simulink model "Lane_Keeping_control_BMW730_auto_sim"  (R2021a)
settings: Solver=FixedStepAuto  StartTime=0.0  StopTime=time  FixedStep=step_size  RelTol=1e-3
values from neighbouring files (symbols this model uses):
  alpha = cf/m+cr/m    (= 169.206008584)    [Dynamic_steering.m]    (also in Dynamic_steering_control_5_1.m; Dynamic_steering_control_5_1_cycle.m; Lane_Keeping_control_BMW730.m)
  alpha_r = alpha    (= 169.206008584)    [Lane_Keeping_control_BMW730.m]
  b1 = cf/m    (= 54.5064377682)    [Dynamic_steering.m]    (also in Dynamic_steering_control_5_1.m; Dynamic_steering_control_5_1_cycle.m; Lane_Keeping_control_BMW730.m)
  b1_r = b1    (= 54.5064377682)    [Lane_Keeping_control_BMW730.m]
  b2 = cf*lf/J    (= 41.9857690203)    [Dynamic_steering.m]    (also in Dynamic_steering_control_5_1.m; Dynamic_steering_control_5_1_cycle.m; Lane_Keeping_control_BMW730.m)
  b2_r = b2    (= 41.9857690203)    [Lane_Keeping_control_BMW730.m]
  beta = -cf*lf+cr*lr    (= 128800)    [Dynamic_steering.m]    (also in Dynamic_steering_control_5_1.m; Dynamic_steering_control_5_1_cycle.m; Lane_Keeping_control_BMW730.m)
  beta_r = beta    (= 128800)    [Lane_Keeping_control_BMW730.m]
  dC = double(dC)    [HM8_Youla.m]    (also in Lane_Keeping_control_BMW730.m)
  gamma = 0.01    [Cart_pendulum.m]    (also in Dynamic_steering.m = 165.348461959; Dynamic_steering_control_5_1.m = 165.348461959; Dynamic_steering_control_5_1_cycle.m = 165.348461959; Lane_Keeping_control_BMW730.m = 165.348461959)
  gamma_r = gamma    (= 165.348461959)    [Lane_Keeping_control_BMW730.m]
  J = 100    [Cart_pendulum.m]    (also in Dynamic_steering.m = 3654; Dynamic_steering_control_5_1.m = 3654; Dynamic_steering_control_5_1_cycle.m = 3654; Lane_Keeping_control_BMW730.m = 3654)
  kd = -1    [Lane_Keeping_control_BMW730.m]
  kI2 = -0.01    [Lane_Keeping_control_BMW730.m]
  kI3 = -0.1    [Lane_Keeping_control_BMW730.m]
  kP2 = -10    [Lane_Keeping_control_BMW730.m]
  m = 50    [Active_suspension_with_control_2.m]    (also in Cart_pendulum.m = 80; Dynamic_steering.m = 1864; Dynamic_steering_control_5_1.m = 1864; Dynamic_steering_control_5_1_cycle.m = 1864)
  nC = double(nC)    [HM8_Youla.m]    (also in Lane_Keeping_control_BMW730.m)
  r = 100    [Lane_Keeping_control_BMW730.m]
  V = Vzf1(2)    [Dynamic_steering.m]    (also in Dynamic_steering_control_5_1.m = 33.3333333333; Dynamic_steering_control_5_1_cycle.m = ( V0/3.6 )*( 1+ i/100 ); Lane_Keeping_control_BMW730.m = 17)
  vy_0 = 2    [Dynamic_steering_control_5_1.m]    (also in Dynamic_steering_control_5_1_cycle.m; Lane_Keeping_control_BMW730.m = 0)
  vy_r0 = 0    [Lane_Keeping_control_BMW730.m]
libraries: simulink x3
settings Model: Creator=Gerardo  LastModifiedBy=adith
settings SolverCC: AlgebraicLoopSolver=TrustRegion
settings DataIOCC: ReturnWorkspaceOutputs=off
settings DebuggingCC: SFMachineParentedDataDiag=warning  ArithmeticOperatorsInVariantConditions=warning
settings SFSimCC: CustomCodeUndefinedFunction=UseInterfaceOnly

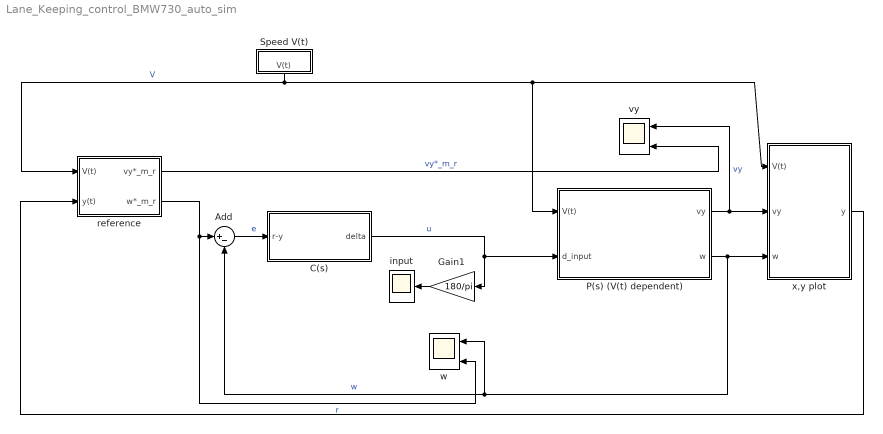
== system Lane_Keeping_control_BMW730_auto_sim ==
  Add : Sum  Inputs=|+-
  C(s) : Subsystem
  Gain1 : Gain  Gain=180/pi
  P(s) (V(t) dependent) : Subsystem
  Speed V(t) : Subsystem
  input : Scope
  reference : Subsystem
  vy : Scope  NumInputPorts=2
  w : Scope  NumInputPorts=2
  x,y plot : Subsystem
  wires:
  C(s)/1(delta) -> P(s) (V(t) dependent)/2(d_input), Gain1/1  "u"
  Add/1 -> C(s)/1(r-y)  "e"
  P(s) (V(t) dependent)/2(w) -> w/1, Add/2, x,y plot/3(w)  "w"
  reference/2(w*_m_r) -> w/2, Add/1  "r"
  P(s) (V(t) dependent)/1(vy) -> x,y plot/2(vy), vy/1  "vy"
  reference/1(vy*_m_r) -> vy/2  "vy*_m_r"
  Speed V(t)/1(V(t)) -> reference/1(V(t)), P(s) (V(t) dependent)/1(V(t)), x,y plot/1(V(t))  "V"
  Gain1/1 -> input/1
  x,y plot/1(y) -> reference/2(y(t))

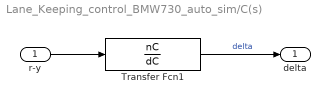
== system Lane_Keeping_control_BMW730_auto_sim/C(s) ==
  r-y : Inport
  Transfer Fcn1 : TransferFcn  Numerator=nC  Denominator=dC
  delta : Outport  VectorParamsAs1DForOutWhenUnconnected=off
  wires:
  Transfer Fcn1/1 -> delta/1  "delta"
  r-y/1 -> Transfer Fcn1/1

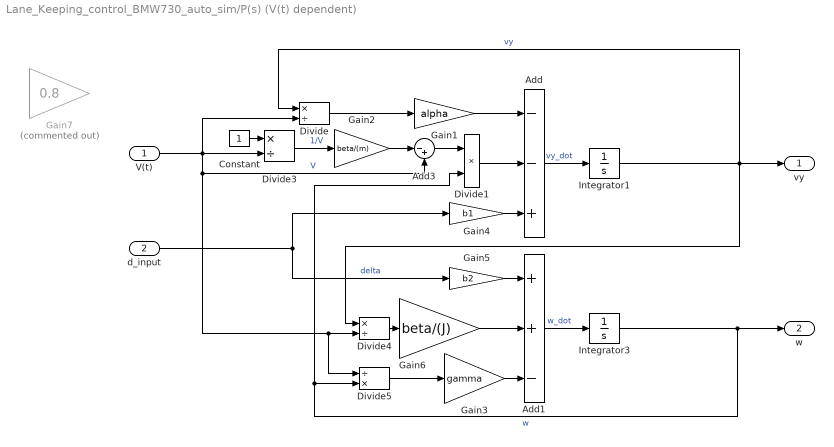
== system Lane_Keeping_control_BMW730_auto_sim/P(s) (V(t) dependent) ==
  V(t) : Inport
  d_input : Inport  Port=2
  Add : Sum  Inputs=--+
  Add1 : Sum  Inputs=++-
  Add3 : Sum  Inputs=|-+
  Constant : Constant
  Divide : Product  Inputs=*/
  Divide1 : Product  Inputs=**
  Divide3 : Product  Inputs=*/
  Divide4 : Product  Inputs=*/
  Divide5 : Product  Inputs=/*
  Gain1 : Gain  Gain=alpha
  Gain2 : Gain  Gain=beta/(m)
  Gain3 : Gain  Gain=gamma
  Gain4 : Gain  Gain=b1
  Gain5 : Gain  Gain=b2
  Gain6 : Gain  Gain=beta/(J)
  Gain7 : Gain  Commented=on  Gain=0.8
  Integrator1 : Integrator  InitialCondition=vy_0
  Integrator3 : Integrator
  vy : Outport  VectorParamsAs1DForOutWhenUnconnected=off
  w : Outport  Port=2  VectorParamsAs1DForOutWhenUnconnected=off
  wires:
  Gain3/1 -> Add1/3
  Add/1 -> Integrator1/1  "vy_dot"
  Add1/1 -> Integrator3/1  "w_dot"
  Gain1/1 -> Add/1
  Gain5/1 -> Add1/1
  Gain4/1 -> Add/3
  Gain2/1 -> Add3/1
  Integrator1/1 -> Divide4/1, Divide/1, vy/1  "vy"
  Divide5/1 -> Gain3/1
  V(t)/1 -> Divide3/2, Divide5/1, Divide4/2, Add3/2, Divide/2  "V"
  Divide3/1 -> Gain2/1  "1/V"
  d_input/1 -> Gain4/1, Gain5/1  "delta"
  Divide4/1 -> Gain6/1
  Gain6/1 -> Add1/2
  Divide1/1 -> Add/2
  Divide/1 -> Gain1/1
  Integrator3/1 -> Divide5/2, Divide1/2, w/1  "w"
  Constant/1 -> Divide3/1
  Add3/1 -> Divide1/1

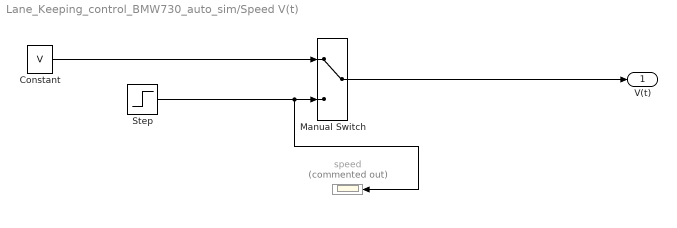
== system Lane_Keeping_control_BMW730_auto_sim/Speed V(t) ==
  Constant : Constant  Value=V
  Manual Switch : ManualSwitch
  Step : Step  Time=7.5  Before=V  After=V*0.85  SampleTime=0
  speed : Scope  Commented=on
  V(t) : Outport  VectorParamsAs1DForOutWhenUnconnected=off
  wires:
  Constant/1 -> Manual Switch/1
  Step/1 -> speed/1, Manual Switch/2
  Manual Switch/1 -> V(t)/1

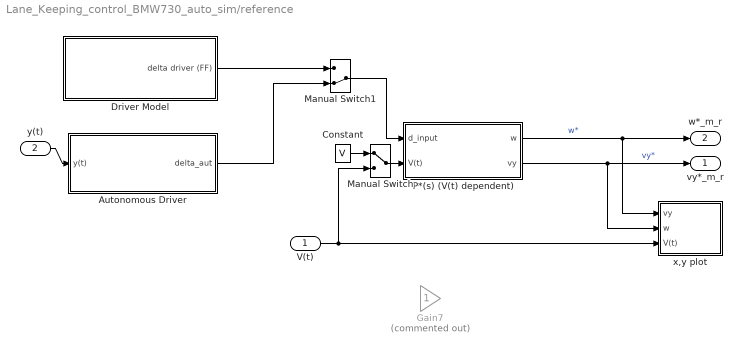
== system Lane_Keeping_control_BMW730_auto_sim/reference ==
  V(t) : Inport
  y(t) : Inport  Port=2
  Autonomous Driver : Subsystem
  Constant : Constant  Value=V
  Driver Model : Subsystem
  Gain7 : Gain  Commented=on
  Manual Switch : ManualSwitch
  Manual Switch1 : ManualSwitch  CurrentSetting=0
  P*(s) (V(t) dependent) : Subsystem
  x,y plot : Subsystem
  vy*_m_r : Outport  VectorParamsAs1DForOutWhenUnconnected=off
  w*_m_r : Outport  Port=2  VectorParamsAs1DForOutWhenUnconnected=off
  wires:
  P*(s) (V(t) dependent)/1(w) -> x,y plot/1(vy), w*_m_r/1  "w*"
  P*(s) (V(t) dependent)/2(vy) -> x,y plot/2(w), vy*_m_r/1  "vy*"
  Manual Switch/1 -> P*(s) (V(t) dependent)/2(V(t))
  Constant/1 -> Manual Switch/1
  V(t)/1 -> Manual Switch/2, x,y plot/3(V(t))
  Manual Switch1/1 -> P*(s) (V(t) dependent)/1(d_input)
  Driver Model/1(delta driver (FF)) -> Manual Switch1/1
  Autonomous Driver/1(delta_aut) -> Manual Switch1/2
  y(t)/1 -> Autonomous Driver/1(y(t))

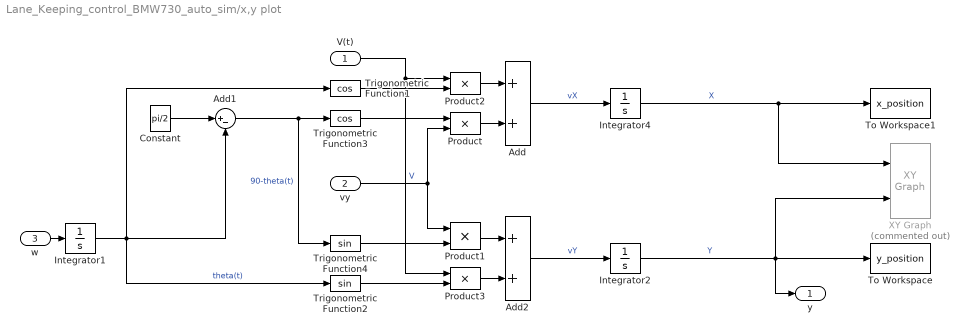
== system Lane_Keeping_control_BMW730_auto_sim/x,y plot ==
  V(t) : Inport
  vy : Inport  Port=2
  w : Inport  Port=3
  Add : Sum
  Add1 : Sum  Inputs=|+-
  Add2 : Sum
  Constant : Constant  Value=pi/2
  Integrator1 : Integrator
  Integrator2 : Integrator
  Integrator4 : Integrator
  Product{,1..3} (4 alike) : Product
  To Workspace : ToWorkspace  VariableName=y_position  SampleTime=-1
      settings: Save2DSignal=2-D array (concatenate along first dimension)
  To Workspace1 : ToWorkspace  VariableName=x_position  SampleTime=-1
      settings: Save2DSignal=2-D array (concatenate along first dimension)
  Trigonometric Function1 : Trigonometry  Operator=cos
  Trigonometric Function2 : Trigonometry
  Trigonometric Function3 : Trigonometry  Operator=cos
  Trigonometric Function4 : Trigonometry
  XY Graph : simulink/Sinks/XY Graph  Commented=on  xmin=-1000  xmax=1000  ymin=-50  ymax=50  st=-1
  y : Outport  VectorParamsAs1DForOutWhenUnconnected=off
  wires:
  Trigonometric Function4/1 -> Product1/2
  Trigonometric Function3/1 -> Product/1
  Product1/1 -> Add2/1
  Trigonometric Function2/1 -> Product3/2
  Add2/1 -> Integrator2/1  "vY"
  Trigonometric Function1/1 -> Product2/2
  Product/1 -> Add/2
  Add1/1 -> Trigonometric Function3/1, Trigonometric Function4/1  "90-theta(t)"
  Integrator1/1 -> Trigonometric Function1/1, Trigonometric Function2/1, Add1/2  "theta(t)"
  w/1 -> Integrator1/1
  Constant/1 -> Add1/1
  Add/1 -> Integrator4/1  "vX"
  Integrator4/1 -> XY Graph/1, To Workspace1/1  "X"
  vy/1 -> Product/2, Product1/1
  Integrator2/1 -> y/1, To Workspace/1, XY Graph/2  "Y"
  Product2/1 -> Add/1
  V(t)/1 -> Product3/1, Product2/1  "V"
  Product3/1 -> Add2/2

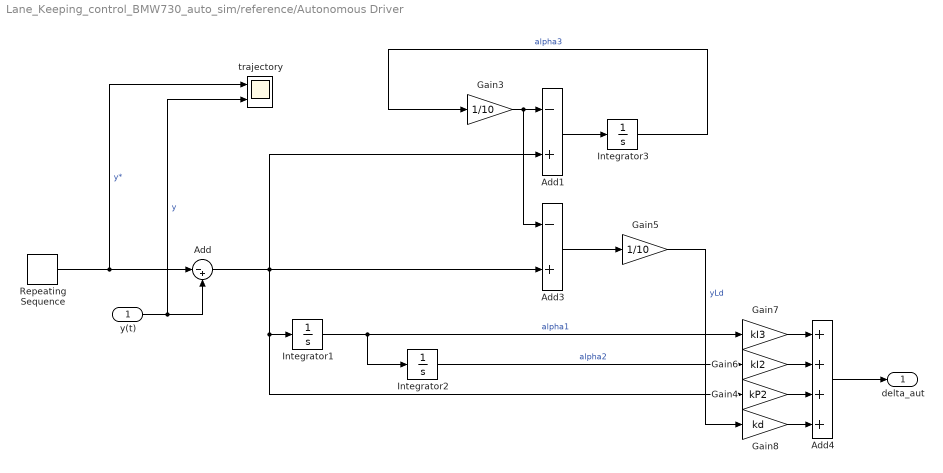
== system Lane_Keeping_control_BMW730_auto_sim/reference/Autonomous Driver ==
  y(t) : Inport
  Add : Sum  Inputs=|-+
  Add1 : Sum  Inputs=-+
  Add3 : Sum  Inputs=-+
  Add4 : Sum  Inputs=++++
  Gain3 : Gain  Gain=1/10
  Gain4 : Gain  Gain=kP2
  Gain5 : Gain  Gain=1/10
  Gain6 : Gain  Gain=kI2
  Gain7 : Gain  Gain=kI3
  Gain8 : Gain  Gain=kd
  Integrator1 : Integrator
  Integrator2 : Integrator
  Integrator3 : Integrator
  Repeating Sequence : simulink/Sources/Repeating Sequence  rep_seq_t=t  rep_seq_y=y_position
  trajectory : Scope  NumInputPorts=2
  delta_aut : Outport  VectorParamsAs1DForOutWhenUnconnected=off
  wires:
  Repeating Sequence/1 -> trajectory/1, Add/1  "y*"
  y(t)/1 -> Add/2, trajectory/2  "y"
  Integrator1/1 -> Gain7/1, Integrator2/1  "alpha1"
  Integrator2/1 -> Gain6/1  "alpha2"
  Integrator3/1 -> Gain3/1  "alpha3"
  Add1/1 -> Integrator3/1
  Add3/1 -> Gain5/1
  Gain3/1 -> Add3/1, Add1/1
  Add/1 -> Add1/2, Add3/2, Gain4/1, Integrator1/1
  Gain5/1 -> Gain8/1  "yLd"
  Gain7/1 -> Add4/1
  Gain6/1 -> Add4/2
  Gain4/1 -> Add4/3
  Gain8/1 -> Add4/4
  Add4/1 -> delta_aut/1

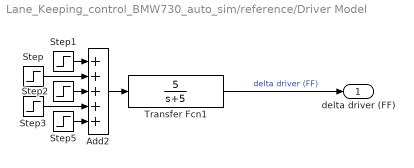
== system Lane_Keeping_control_BMW730_auto_sim/reference/Driver Model ==
  Add2 : Sum  Inputs=+++++
  Step : Step  Time=(100+0.025*(2*pi*r))/V  After=V/(r)  SampleTime=0
  Step1 : Step  Time=100/V  After=-V/(r)  SampleTime=0
  Step2 : Step  Time=(100+0.025*(2*pi*r))/V  After=V/(r)  SampleTime=0
  Step3 : Step  Time=(100+0.075*(2*pi*r))/V  After=-2*V/(r)  SampleTime=0
  Step5 : Step  Time=(100+0.1*(2*pi*r))/V  After=V/(r)  SampleTime=0
  Transfer Fcn1 : TransferFcn  Numerator=[5]  Denominator=[1 5]
  delta driver (FF) : Outport  VectorParamsAs1DForOutWhenUnconnected=off
  wires:
  Transfer Fcn1/1 -> delta driver (FF)/1  "delta driver (FF)"
  Step3/1 -> Add2/4
  Step/1 -> Add2/2
  Step2/1 -> Add2/3
  Add2/1 -> Transfer Fcn1/1
  Step5/1 -> Add2/5
  Step1/1 -> Add2/1

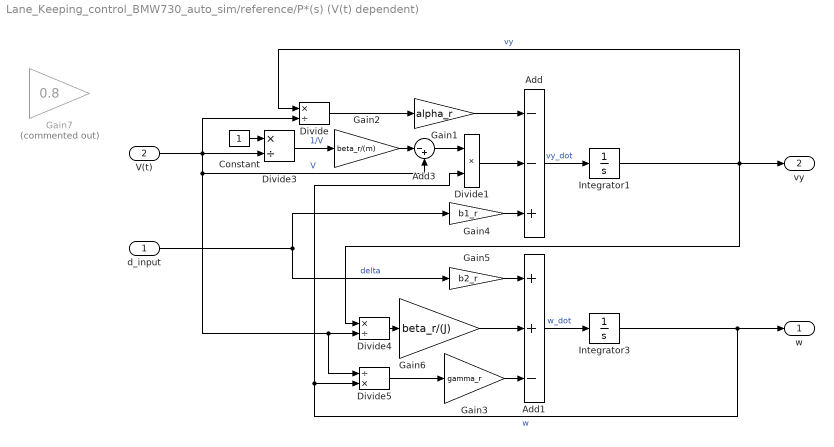
== system Lane_Keeping_control_BMW730_auto_sim/reference/P*(s) (V(t) dependent) ==
  d_input : Inport
  V(t) : Inport  Port=2
  Add : Sum  Inputs=--+
  Add1 : Sum  Inputs=++-
  Add3 : Sum  Inputs=|-+
  Constant : Constant
  Divide : Product  Inputs=*/
  Divide1 : Product  Inputs=**
  Divide3 : Product  Inputs=*/
  Divide4 : Product  Inputs=*/
  Divide5 : Product  Inputs=/*
  Gain1 : Gain  Gain=alpha_r
  Gain2 : Gain  Gain=beta_r/(m)
  Gain3 : Gain  Gain=gamma_r
  Gain4 : Gain  Gain=b1_r
  Gain5 : Gain  Gain=b2_r
  Gain6 : Gain  Gain=beta_r/(J)
  Gain7 : Gain  Commented=on  Gain=0.8
  Integrator1 : Integrator  InitialCondition=vy_r0
  Integrator3 : Integrator
  w : Outport  VectorParamsAs1DForOutWhenUnconnected=off
  vy : Outport  Port=2  VectorParamsAs1DForOutWhenUnconnected=off
  wires:
  Gain3/1 -> Add1/3
  Add/1 -> Integrator1/1  "vy_dot"
  Add1/1 -> Integrator3/1  "w_dot"
  Gain1/1 -> Add/1
  Gain5/1 -> Add1/1
  Gain4/1 -> Add/3
  Gain2/1 -> Add3/1
  Integrator1/1 -> Divide4/1, Divide/1, vy/1  "vy"
  Divide5/1 -> Gain3/1
  V(t)/1 -> Divide3/2, Divide5/1, Divide4/2, Add3/2, Divide/2  "V"
  Divide3/1 -> Gain2/1  "1/V"
  d_input/1 -> Gain4/1, Gain5/1  "delta"
  Divide4/1 -> Gain6/1
  Gain6/1 -> Add1/2
  Divide1/1 -> Add/2
  Divide/1 -> Gain1/1
  Integrator3/1 -> Divide5/2, Divide1/2, w/1  "w"
  Constant/1 -> Divide3/1
  Add3/1 -> Divide1/1

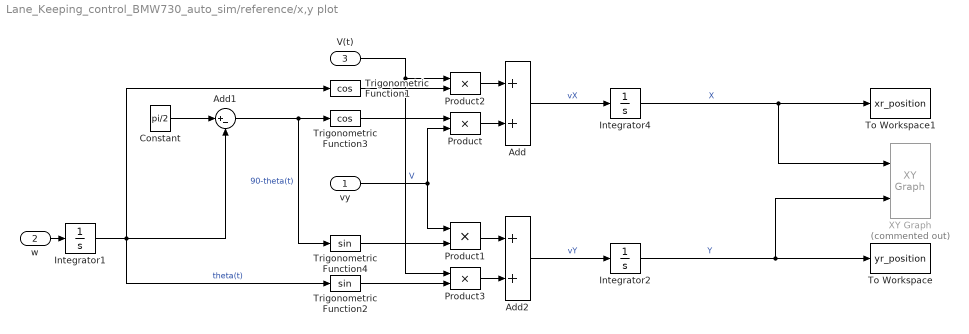
== system Lane_Keeping_control_BMW730_auto_sim/reference/x,y plot ==
  vy : Inport
  w : Inport  Port=2
  V(t) : Inport  Port=3
  Add : Sum
  Add1 : Sum  Inputs=|+-
  Add2 : Sum
  Constant : Constant  Value=pi/2
  Integrator1 : Integrator
  Integrator2 : Integrator
  Integrator4 : Integrator
  Product{,1..3} (4 alike) : Product
  To Workspace : ToWorkspace  VariableName=yr_position  SampleTime=-1
      settings: Save2DSignal=2-D array (concatenate along first dimension)
  To Workspace1 : ToWorkspace  VariableName=xr_position  SampleTime=-1
      settings: Save2DSignal=2-D array (concatenate along first dimension)
  Trigonometric Function1 : Trigonometry  Operator=cos
  Trigonometric Function2 : Trigonometry
  Trigonometric Function3 : Trigonometry  Operator=cos
  Trigonometric Function4 : Trigonometry
  XY Graph : simulink/Sinks/XY Graph  Commented=on  xmin=-1000  xmax=1000  ymin=-50  ymax=50  st=-1
  wires:
  Trigonometric Function4/1 -> Product1/2
  Trigonometric Function3/1 -> Product/1
  Product1/1 -> Add2/1
  Trigonometric Function2/1 -> Product3/2
  Add2/1 -> Integrator2/1  "vY"
  Trigonometric Function1/1 -> Product2/2
  Product/1 -> Add/2
  Add1/1 -> Trigonometric Function3/1, Trigonometric Function4/1  "90-theta(t)"
  Integrator1/1 -> Trigonometric Function1/1, Trigonometric Function2/1, Add1/2  "theta(t)"
  w/1 -> Integrator1/1
  Constant/1 -> Add1/1
  Add/1 -> Integrator4/1  "vX"
  Integrator4/1 -> XY Graph/1, To Workspace1/1  "X"
  vy/1 -> Product/2, Product1/1
  Integrator2/1 -> XY Graph/2, To Workspace/1  "Y"
  Product2/1 -> Add/1
  V(t)/1 -> Product3/1, Product2/1  "V"
  Product3/1 -> Add2/2
